simulink model "withoutintegral"  (Simulink 7.3)
settings: Solver=ode45  StartTime=0.0  StopTime=20  RelTol=1e-3
libraries: powerlib x1
settings Model: Creator=HP  LastModifiedBy=Twad1
settings OptimizationCC: ExpressionDepthLimit=128
settings DebuggingCC: UnderspecifiedInitializationDetection=Simplified  MergeDetectMultiDrivingBlocksExec=error  SolverPrmCheckMsg=none  StateNameClashWarn=none  StrictBusMsg=ErrorLevel1
settings CodeAppCC: CustomSymbolStrType=$N$R$M_T
settings GRTTargetCC: TargetFunctionLibrary=NOT IN USE  CombineOutputUpdateFcns=on  CPPClassGenCompliant=on

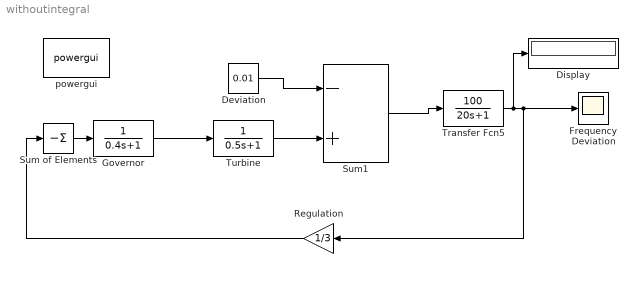
== system withoutintegral ==
  Deviation : Constant  Value=0.01  OutDataType=fixdt(1, 16)  OutScaling=2^0
  Display : Display
  Frequency Deviation : Scope
      settings: SaveName=withoutintegral
  Governor : TransferFcn  Denominator=[0.4 1]
  Regulation : Gain  Gain=1/3
  Sum of Elements : Sum  Inputs=-
  Sum1 : Sum  Inputs=-+
  Transfer Fcn5 : TransferFcn  Numerator=[100]  Denominator=[20 1]
  Turbine : TransferFcn  Denominator=[0.5 1]
  powergui : powerlib/powergui  Priority=1  SystemSampleTime=-1  SimulationMode=Continuous  SampleTime=50e-6  frequency=60  SPID=off  DisableSnubberDevices=off  DisableRonSwitches=off  DisableVfSwitches=off  SwTol=0  Interpol=off  frequencyindice=60  echomessages=off  HookPort=off  DisplayEquations=off  FunctionMessages=off  EnableUseOfTLC=off  x0status=blocks  RestoreLinks=warning  Frange=[0:2:500]  Ylog=off  Xlog=on  ShowGrid=off  save=off  variable=ZData  structure=0  ZoomFFT=off  StartTime=0.0  cycles=1  DisplayStyle=1  fundamental=60  FreqAxis=off  MaxFrequency=1000  frequencyindicesteady=1  RmsSteady=1  display=off  Ts=100  methode=off
  wires:
  Sum of Elements/1 -> Governor/1
  Governor/1 -> Turbine/1
  Turbine/1 -> Sum1/2
  Sum1/1 -> Transfer Fcn5/1
  Regulation/1 -> Sum of Elements/1
  Deviation/1 -> Sum1/1
  Transfer Fcn5/1 -> Frequency Deviation/1, Regulation/1, Display/1
